simulink model "D4_simulink"  (R2015a)
settings: Solver=ode45  StartTime=0.0  StopTime=0.8  RelTol=1e-3
settings Model: Creator=declangilmour  LastModifiedBy=declangilmour

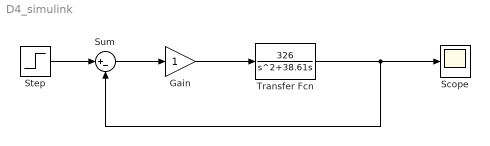
== system D4_simulink ==
  Gain : Gain
  Scope : Scope
  Step : Step  Time=0  SampleTime=0.001
  Sum : Sum  Inputs=|+-
  Transfer Fcn : TransferFcn  Numerator=[326]  Denominator=[1 38.61 0]
  wires:
  Step/1 -> Sum/1
  Sum/1 -> Gain/1
  Gain/1 -> Transfer Fcn/1
  Transfer Fcn/1 -> Sum/2, Scope/1
